simulink model "PVPanelAnn"  (R2018a)
settings: Solver=FixedStepDiscrete  StartTime=0.0  StopTime=10.0  FixedStep=10e-6  RelTol=1e-3
libraries: neural x37, powerlib x9, simulink x1, re_lib x1, powerlib_meascontrol x1
(part 2 of 2)

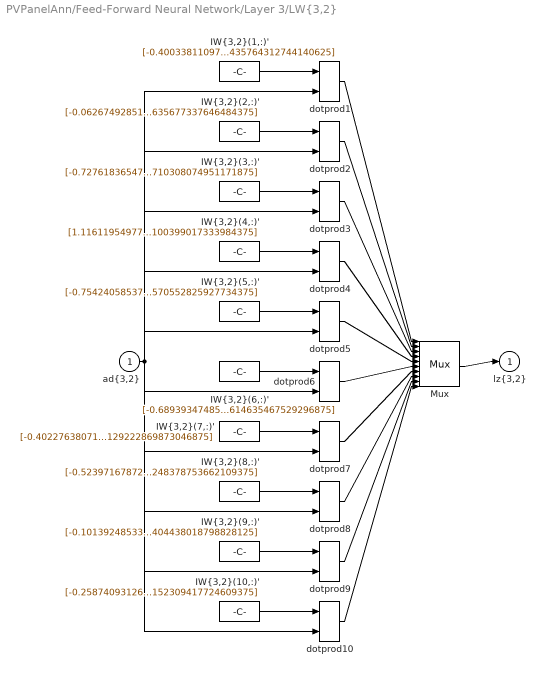
== system PVPanelAnn/Feed-Forward Neural Network/Layer 3/LW{3,2} ==
  "ad{3,2}" : Inport  PortDimensions=10
      mask Display: e = 0.06;c1 = [120 230 180]/255;c2 = ([120 230 180]+0)/(256+128);c3 = ([120 230 180]+128)/(256+128);patch([0 1 1 0],[0 0 1 1],c1);patch([0 1 1 1-e 1-e 0+e],[0 0 1 1-e 0+e 0+e],c2);patch([0 0 1 1-e 0+e 0+e],[0 1 1 1-e 1-e 0+e],c3);plot([0 1 1 0 0],[0 0 1 1 0]);
  "IW{3,2}(1,:)'" : Constant  Value=[-0.400338110971180161090643423449364490807056427001953125;0.8694233749757442897276860094279982149600982666015625;-0.38254126374922148290380619073403067886829376220703125;-0.89989166561537192734476775513030588626861572265625;0.278829451887158186185189379102666862308979034423828125;-0.477614720844293294543803085616673342883586883544921875;0.782722583498746349306429692660458385944366455078125;-0.1489556546810286707938075778656639158725738525390625;0.059816683163513205412353812562287203036248683929443359375;0.53686587401000240848958355854847468435764312744140625]
      mask Display: e = 0.06;c1 = [120 150 230]/255;c2 = ([120 150 230]+0)/383;c3 = ([120 150 230]+128)/383;patch([0 1 1 0],[0 0 1 1],c1);patch([0 1 1 1-e 1-e 0+e],[0 0 1 1-e 0+e 0+e],c2);patch([0 0 1 1-e 0+e 0+e],[0 1 1 1-e 1-e 0+e],c3);plot([0 1 1 0 0],[0 0 1 1 0]);disp('weights');
  "IW{3,2}(10,:)'" : Constant  Value=[-0.25874093126525021801853654324077069759368896484375;0.7991198107052890353685370428138412535190582275390625;-0.60785378763352515552043087154743261635303497314453125;0.67466951980289902035536897528800182044506072998046875;-0.05023303892871074094461647518983227200806140899658203125;-0.70654425351903704655143201307510025799274444580078125;-0.62460753938001101204235965269617736339569091796875;-0.355064856608762635659104489604942500591278076171875;0.221181694480177715167457108691451139748096466064453125;0.667296540881385791266211526817642152309417724609375]
      mask Display: e = 0.06;c1 = [120 150 230]/255;c2 = ([120 150 230]+0)/383;c3 = ([120 150 230]+128)/383;patch([0 1 1 0],[0 0 1 1],c1);patch([0 1 1 1-e 1-e 0+e],[0 0 1 1-e 0+e 0+e],c2);patch([0 0 1 1-e 0+e 0+e],[0 1 1 1-e 1-e 0+e],c3);plot([0 1 1 0 0],[0 0 1 1 0]);disp('weights');
  "IW{3,2}(2,:)'" : Constant  Value=[-0.06267492851838905865147211216026335023343563079833984375;0.96438363351918088284264740650542080402374267578125;0.33336077948906350787439123450894840061664581298828125;0.233821609542878727783232761794351972639560699462890625;-0.1905546347087753444871083274847478605806827545166015625;-0.440971048882607019603341313995770178735256195068359375;0.841553566300655031540145500912331044673919677734375;-0.93690184843638479872396374048548750579357147216796875;0.440539283796392788783435889854445122182369232177734375;-0.28385327720384212479842744869529269635677337646484375]
      mask Display: e = 0.06;c1 = [120 150 230]/255;c2 = ([120 150 230]+0)/383;c3 = ([120 150 230]+128)/383;patch([0 1 1 0],[0 0 1 1],c1);patch([0 1 1 1-e 1-e 0+e],[0 0 1 1-e 0+e 0+e],c2);patch([0 0 1 1-e 0+e 0+e],[0 1 1 1-e 1-e 0+e],c3);plot([0 1 1 0 0],[0 0 1 1 0]);disp('weights');
  "IW{3,2}(3,:)'" : Constant  Value=[-0.72761836547458458301917971766670234501361846923828125;-0.8559318673066378391212083442951552569866180419921875;0.1719462870202414228604226309471414424479007720947265625;0.7954631198540493830506648009759373962879180908203125;-0.562181608831226586886486984440125524997711181640625;0.406623092640918393225746285679633729159832000732421875;0.57767355304976752972123676954652182757854461669921875;-0.0289588297688909424021375116353738121688365936279296875;0.042983907918941077763719249560381285846233367919921875;-0.722611849358983260316335872630588710308074951171875]
      mask Display: e = 0.06;c1 = [120 150 230]/255;c2 = ([120 150 230]+0)/383;c3 = ([120 150 230]+128)/383;patch([0 1 1 0],[0 0 1 1],c1);patch([0 1 1 1-e 1-e 0+e],[0 0 1 1-e 0+e 0+e],c2);patch([0 0 1 1-e 0+e 0+e],[0 1 1 1-e 1-e 0+e],c3);plot([0 1 1 0 0],[0 0 1 1 0]);disp('weights');
  "IW{3,2}(4,:)'" : Constant  Value=[1.1161195497796676523449832529877312481403350830078125;0.540115810105209703806394827552139759063720703125;0.0754497771213483436891777955679572187364101409912109375;0.397275726061327549842872031149454414844512939453125;-0.1455710422441299500828648660899489186704158782958984375;-0.5200901505603681140854632758419029414653778076171875;-0.5369572880646129586779125020257197320461273193359375;-0.07975679373411802275395388051038025878369808197021484375;0.74177364884870577999009810810093767940998077392578125;-0.5327395207513434538526553296833299100399017333984375]
      mask Display: e = 0.06;c1 = [120 150 230]/255;c2 = ([120 150 230]+0)/383;c3 = ([120 150 230]+128)/383;patch([0 1 1 0],[0 0 1 1],c1);patch([0 1 1 1-e 1-e 0+e],[0 0 1 1-e 0+e 0+e],c2);patch([0 0 1 1-e 0+e 0+e],[0 1 1 1-e 1-e 0+e],c3);plot([0 1 1 0 0],[0 0 1 1 0]);disp('weights');
  "IW{3,2}(5,:)'" : Constant  Value=[-0.7542405853778022528643987243412993848323822021484375;-0.5750641717326872015547678529401309788227081298828125;0.45675449871804107981887455025571398437023162841796875;-0.70591554585961358014856159570626914501190185546875;-0.142844506429621542764607511344365775585174560546875;0.6866296912063611923571215811534784734249114990234375;0.2291978421503099438982786750784725882112979888916015625;0.471857918421606015169089687333325855433940887451171875;0.44531981015061006257127473872969858348369598388671875;-0.8057381672616423795574291943921707570552825927734375]
      mask Display: e = 0.06;c1 = [120 150 230]/255;c2 = ([120 150 230]+0)/383;c3 = ([120 150 230]+128)/383;patch([0 1 1 0],[0 0 1 1],c1);patch([0 1 1 1-e 1-e 0+e],[0 0 1 1-e 0+e 0+e],c2);patch([0 0 1 1-e 0+e 0+e],[0 1 1 1-e 1-e 0+e],c3);plot([0 1 1 0 0],[0 0 1 1 0]);disp('weights');
  "IW{3,2}(6,:)'" : Constant  Value=[-0.689393474856548227336361378547735512256622314453125;-0.157679116852917022839619676233269274234771728515625;0.22926574731427551423479371806024573743343353271484375;-0.2395800234598070288516424852787167765200138092041015625;-0.50151096106986958744755611405707895755767822265625;0.87048237868018241147893832021509297192096710205078125;-0.65886992906040575679327275793184526264667510986328125;0.1694671393184606633663946695378399454057216644287109375;0.93997148325695578652272388353594578802585601806640625;-0.364985171235056415905972926339018158614635467529296875]
      mask Display: e = 0.06;c1 = [120 150 230]/255;c2 = ([120 150 230]+0)/383;c3 = ([120 150 230]+128)/383;patch([0 1 1 0],[0 0 1 1],c1);patch([0 1 1 1-e 1-e 0+e],[0 0 1 1-e 0+e 0+e],c2);patch([0 0 1 1-e 0+e 0+e],[0 1 1 1-e 1-e 0+e],c3);plot([0 1 1 0 0],[0 0 1 1 0]);disp('weights');
  "IW{3,2}(7,:)'" : Constant  Value=[-0.40227638071945992503941624818253330886363983154296875;0.16825842999753015671871025915606878697872161865234375;-1.2606347161486863850399231523624621331691741943359375;-0.08113382646277979282078973710667924024164676666259765625;0.239011286941343492618017307904665358364582061767578125;0.846145630063546150267939083278179168701171875;-0.354422385063330291909977631803485564887523651123046875;0.54256443695439993124551847358816303312778472900390625;0.1393133748143687566933834887095144949853420257568359375;-0.2454285722041255890513156145971152000129222869873046875]
      mask Display: e = 0.06;c1 = [120 150 230]/255;c2 = ([120 150 230]+0)/383;c3 = ([120 150 230]+128)/383;patch([0 1 1 0],[0 0 1 1],c1);patch([0 1 1 1-e 1-e 0+e],[0 0 1 1-e 0+e 0+e],c2);patch([0 0 1 1-e 0+e 0+e],[0 1 1 1-e 1-e 0+e],c3);plot([0 1 1 0 0],[0 0 1 1 0]);disp('weights');
  "IW{3,2}(8,:)'" : Constant  Value=[-0.52397167872600458604637196913245134055614471435546875;0.76536297362834948554421998778707347810268402099609375;-0.6457196853664035618436400909558869898319244384765625;0.8302131454891747974755844552419148385524749755859375;-0.44704173051811080252804231349728070199489593505859375;-0.251517420360679200275200173564371652901172637939453125;-0.30659722985713511178573753568343818187713623046875;-0.81742879479941221720906696646125055849552154541015625;-0.290069915060020611097257869914756156504154205322265625;0.048128693832811063335608281477107084356248378753662109375]
      mask Display: e = 0.06;c1 = [120 150 230]/255;c2 = ([120 150 230]+0)/383;c3 = ([120 150 230]+128)/383;patch([0 1 1 0],[0 0 1 1],c1);patch([0 1 1 1-e 1-e 0+e],[0 0 1 1-e 0+e 0+e],c2);patch([0 0 1 1-e 0+e 0+e],[0 1 1 1-e 1-e 0+e],c3);plot([0 1 1 0 0],[0 0 1 1 0]);disp('weights');
  "IW{3,2}(9,:)'" : Constant  Value=[-0.10139248533040980115860207888545119203627109527587890625;-0.165059759445960130275210531181073747575283050537109375;1.0033078220325382101663080902653746306896209716796875;-0.7201051375730376236106167198158800601959228515625;-0.05566906382077464743307615435696789063513278961181640625;0.331778491654150020639946205847081728279590606689453125;-0.536904368640737317264211014844477176666259765625;-0.935391755860383700138527274248190224170684814453125;-0.63844921680500743566000210194033570587635040283203125;-0.04594261295088748753290275317340274341404438018798828125]
      mask Display: e = 0.06;c1 = [120 150 230]/255;c2 = ([120 150 230]+0)/383;c3 = ([120 150 230]+128)/383;patch([0 1 1 0],[0 0 1 1],c1);patch([0 1 1 1-e 1-e 0+e],[0 0 1 1-e 0+e 0+e],c2);patch([0 0 1 1-e 0+e 0+e],[0 1 1 1-e 1-e 0+e],c3);plot([0 1 1 0 0],[0 0 1 1 0]);disp('weights');
  Mux : Mux  Inputs=10
      mask Display: e = 0.06;c1 = [120 150 230]/255;c2 = ([120 150 230]+0)/383;c3 = ([120 150 230]+128)/383;patch([0 1 1 0],[0 0 1 1],c1);patch([0 1 1 1-e 1-e 0+e],[0 0 1 1-e 0+e 0+e],c2);patch([0 0 1 1-e 0+e 0+e],[0 1 1 1-e 1-e 0+e],c3);plot([0 1 1 0 0],[0 0 1 1 0]);disp('Mux');
  dotprod{1..10} (10 alike) : neural/Weight Functions/dotprod
  "lz{3,2}" : Outport
      mask Display: e = 0.06;c1 = [120 230 180]/255;c2 = ([120 230 180]+0)/(256+128);c3 = ([120 230 180]+128)/(256+128);patch([0 1 1 0],[0 0 1 1],c1);patch([0 1 1 1-e 1-e 0+e],[0 0 1 1-e 0+e 0+e],c2);patch([0 0 1 1-e 0+e 0+e],[0 1 1 1-e 1-e 0+e],c3);plot([0 1 1 0 0],[0 0 1 1 0]);
  wires:
  "IW{3,2}(1,:)'"/1 -> dotprod1/1
  "ad{3,2}"/1 -> dotprod1/2, dotprod2/2, dotprod3/2, dotprod4/2, dotprod5/2, dotprod6/2, dotprod7/2, dotprod8/2, dotprod9/2, dotprod10/2
  dotprod1/1 -> Mux/1
  "IW{3,2}(2,:)'"/1 -> dotprod2/1
  dotprod2/1 -> Mux/2
  "IW{3,2}(3,:)'"/1 -> dotprod3/1
  dotprod3/1 -> Mux/3
  "IW{3,2}(4,:)'"/1 -> dotprod4/1
  dotprod4/1 -> Mux/4
  "IW{3,2}(5,:)'"/1 -> dotprod5/1
  dotprod5/1 -> Mux/5
  "IW{3,2}(6,:)'"/1 -> dotprod6/1
  dotprod6/1 -> Mux/6
  "IW{3,2}(7,:)'"/1 -> dotprod7/1
  dotprod7/1 -> Mux/7
  "IW{3,2}(8,:)'"/1 -> dotprod8/1
  dotprod8/1 -> Mux/8
  "IW{3,2}(9,:)'"/1 -> dotprod9/1
  dotprod9/1 -> Mux/9
  "IW{3,2}(10,:)'"/1 -> dotprod10/1
  dotprod10/1 -> Mux/10
  Mux/1 -> "lz{3,2}"/1

== system PVPanelAnn/Feed-Forward Neural Network/Layer 4/Delays 1 ==
  "p{4}" : Inport  PortDimensions=10
      mask Display: e = 0.06;c1 = [120 230 180]/255;c2 = ([120 230 180]+0)/(256+128);c3 = ([120 230 180]+128)/(256+128);patch([0 1 1 0],[0 0 1 1],c1);patch([0 1 1 1-e 1-e 0+e],[0 0 1 1-e 0+e 0+e],c2);patch([0 0 1 1-e 0+e 0+e],[0 1 1 1-e 1-e 0+e],c3);plot([0 1 1 0 0],[0 0 1 1 0]);
  mux : Mux  Inputs=1
      mask Display: e = 0.06;c1 = [120 150 230]/255;c2 = ([120 150 230]+0)/383;c3 = ([120 150 230]+128)/383;patch([0 1 1 0],[0 0 1 1],c1);patch([0 1 1 1-e 1-e 0+e],[0 0 1 1-e 0+e 0+e],c2);patch([0 0 1 1-e 0+e 0+e],[0 1 1 1-e 1-e 0+e],c3);plot([0 1 1 0 0],[0 0 1 1 0]);disp('Mux')
  "pd{4,3}" : Outport
      mask Display: e = 0.06;c1 = [120 230 180]/255;c2 = ([120 230 180]+0)/(256+128);c3 = ([120 230 180]+128)/(256+128);patch([0 1 1 0],[0 0 1 1],c1);patch([0 1 1 1-e 1-e 0+e],[0 0 1 1-e 0+e 0+e],c2);patch([0 0 1 1-e 0+e 0+e],[0 1 1 1-e 1-e 0+e],c3);plot([0 1 1 0 0],[0 0 1 1 0]);
  wires:
  "p{4}"/1 -> mux/1
  mux/1 -> "pd{4,3}"/1

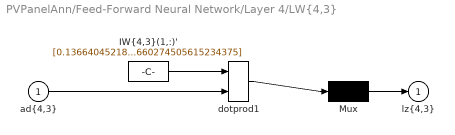
== system PVPanelAnn/Feed-Forward Neural Network/Layer 4/LW{4,3} ==
  "ad{4,3}" : Inport  PortDimensions=10
      mask Display: e = 0.06;c1 = [120 230 180]/255;c2 = ([120 230 180]+0)/(256+128);c3 = ([120 230 180]+128)/(256+128);patch([0 1 1 0],[0 0 1 1],c1);patch([0 1 1 1-e 1-e 0+e],[0 0 1 1-e 0+e 0+e],c2);patch([0 0 1 1-e 0+e 0+e],[0 1 1 1-e 1-e 0+e],c3);plot([0 1 1 0 0],[0 0 1 1 0]);
  "IW{4,3}(1,:)'" : Constant  Value=[0.13664045218554854432824186005746014416217803955078125;1.0536079459361811228035321619245223701000213623046875;0.255406376111833199882283906845259480178356170654296875;0.80375819117225366650103524079895578324794769287109375;-0.413939118201533451379958705729222856462001800537109375;0.456648313605845956875128877072711475193500518798828125;-0.230580537915488215094939050686662085354328155517578125;0.2216538884914461549069386592236696742475032806396484375;0.26536044225056787393413060271996073424816131591796875;-0.9352805815806757294694762094877660274505615234375]
      mask Display: e = 0.06;c1 = [120 150 230]/255;c2 = ([120 150 230]+0)/383;c3 = ([120 150 230]+128)/383;patch([0 1 1 0],[0 0 1 1],c1);patch([0 1 1 1-e 1-e 0+e],[0 0 1 1-e 0+e 0+e],c2);patch([0 0 1 1-e 0+e 0+e],[0 1 1 1-e 1-e 0+e],c3);plot([0 1 1 0 0],[0 0 1 1 0]);disp('weights');
  Mux : Mux  Inputs=1
      mask Display: e = 0.06;c1 = [120 150 230]/255;c2 = ([120 150 230]+0)/383;c3 = ([120 150 230]+128)/383;patch([0 1 1 0],[0 0 1 1],c1);patch([0 1 1 1-e 1-e 0+e],[0 0 1 1-e 0+e 0+e],c2);patch([0 0 1 1-e 0+e 0+e],[0 1 1 1-e 1-e 0+e],c3);plot([0 1 1 0 0],[0 0 1 1 0]);disp('Mux');
  dotprod1 : neural/Weight Functions/dotprod
  "lz{4,3}" : Outport
      mask Display: e = 0.06;c1 = [120 230 180]/255;c2 = ([120 230 180]+0)/(256+128);c3 = ([120 230 180]+128)/(256+128);patch([0 1 1 0],[0 0 1 1],c1);patch([0 1 1 1-e 1-e 0+e],[0 0 1 1-e 0+e 0+e],c2);patch([0 0 1 1-e 0+e 0+e],[0 1 1 1-e 1-e 0+e],c3);plot([0 1 1 0 0],[0 0 1 1 0]);
  wires:
  "IW{4,3}(1,:)'"/1 -> dotprod1/1
  "ad{4,3}"/1 -> dotprod1/2
  dotprod1/1 -> Mux/1
  Mux/1 -> "lz{4,3}"/1
